simulink model "model_QK_SFSVD_ROS"  (Simulink 7.6)
settings: Solver=FixedStepDiscrete  SolverMode=SingleTasking  StartTime=0  StopTime=100  FixedStep=0.01  RelTol=1e-3
values from neighbouring files (symbols this model uses):
  parameter = block.DialogPrm(3).Data    [Kalmangain.m]    (also in init_QK_ROS.m = load('parameter'); statePrediction.m = block.DialogPrm(2).Data)
libraries: PortLib x11, simulink x2, aerolibutil x2
(part 1 of 4)
settings Model: Creator=sendobry  LastModifiedBy=sendobry
settings SolverCC: MaxConsecutiveMinStep=10
settings OptimizationCC: AccelVerboseBuild=on
settings DebuggingCC: ArrayBoundsChecking=warning  UnderspecifiedInitializationDetection=Simplified
settings RTWCC: SystemTargetFile=orocos.tlc  TemplateMakefile=orocos.tmf  Description=Linux Orocos Target  ProcessScript=orocos_make_rtw_hook
settings STFCustomTargetCC: ModelReferenceCompliant=off  GeneratePreprocessorConditionals=Disable all  MatFileLogging=on  SystemTargetFile=orocos.tlc

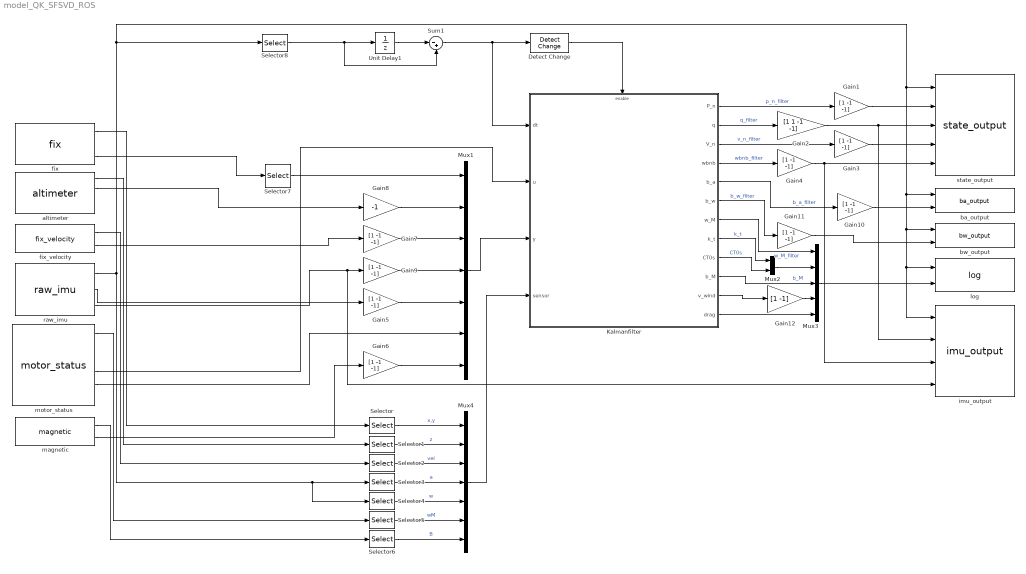
== system model_QK_SFSVD_ROS ==
  Detect Change : simulink/Logic and Bit Operations/Detect Change  SystemSampleTime=-1  vinit=0
  Gain{1,3..7,9..11} (9 alike) : Gain  Gain=[1 -1 -1]
  Gain12 : Gain  Gain=[1 -1]
  Gain2 : Gain  Gain=[1 1 -1 -1]
  Gain8 : Gain  Gain=-1
  Kalmanfilter : Subsystem
  Mux1 : Mux  Inputs=7
  Mux2 : Mux  Inputs=2
  Mux3 : Mux  Inputs=5
  Mux4 : Mux  Inputs=7
  Selector{,1..6,8} (8 alike) : Selector  InputPortWidth=2  IndexOptions=Index vector (dialog)  Indices=2  OutputSizes=1
  Selector7 : Selector  InputPortWidth=3  IndexOptions=Index vector (dialog)  Indices=[1 2]  OutputSizes=1
  Sum1 : Sum  Inputs=|-+
  Unit Delay1 : UnitDelay  SampleTime=-1
  altimeter : PortLib/altimeter  SystemSampleTime=-1
  ba_output : PortLib/ba_output  SystemSampleTime=-1
  bw_output : PortLib/bw_output  SystemSampleTime=-1
  fix : PortLib/fix  SystemSampleTime=-1
  fix_velocity : PortLib/fix_velocity  SystemSampleTime=-1
  imu_output : PortLib/imu_output  SystemSampleTime=-1
  log : PortLib/log  SystemSampleTime=-1
  magnetic : PortLib/magnetic  SystemSampleTime=-1
  motor_status : PortLib/motor_status  SystemSampleTime=-1
  raw_imu : PortLib/raw_imu  SystemSampleTime=-1
  state_output : PortLib/state_output  SystemSampleTime=-1
  wires:
  motor_status/4 -> Kalmanfilter/2(u)
  fix/3 -> Selector7/1
  altimeter/2 -> Gain8/1
  fix_velocity/2 -> Gain7/1
  raw_imu/3 -> Gain9/1, imu_output/4
  raw_imu/2 -> Gain5/1
  magnetic/2 -> Gain6/1
  Mux1/1 -> Kalmanfilter/3(y)
  Mux4/1 -> Kalmanfilter/4(sensor)
  Unit Delay1/1 -> Sum1/1
  Selector/1 -> Mux4/1  "x,y"
  Selector1/1 -> Mux4/2  "z"
  Selector2/1 -> Mux4/3  "vel"
  Selector3/1 -> Mux4/4  "a"
  Selector4/1 -> Mux4/5  "w"
  Selector5/1 -> Mux4/6  "wM"
  Selector6/1 -> Mux4/7  "B"
  fix/1 -> Selector/1
  altimeter/1 -> Selector1/1
  raw_imu/1 -> Selector3/1, Selector4/1, Selector8/1, ba_output/1, bw_output/1, log/1, imu_output/1, state_output/1
  magnetic/1 -> Selector6/1
  fix_velocity/1 -> Selector2/1
  Selector8/1 -> Sum1/2, Unit Delay1/1
  motor_status/1 -> Selector5/1
  Kalmanfilter/1(P_n) -> Gain1/1  "p_n_filter"
  Kalmanfilter/4(wbnb) -> Gain4/1  "wbnb_filter"
  Kalmanfilter/2(q) -> Gain2/1  "q_filter"
  Kalmanfilter/3(V_n) -> Gain3/1  "v_n_filter"
  Gain5/1 -> Mux1/5
  Gain6/1 -> Mux1/7
  Gain7/1 -> Mux1/3
  Gain8/1 -> Mux1/2
  Gain9/1 -> Mux1/4
  Selector7/1 -> Mux1/1
  Kalmanfilter/5(b_a) -> Gain10/1  "b_a_filter"
  Kalmanfilter/6(b_w) -> Gain11/1  "b_w_filter"
  Kalmanfilter/7(w_M) -> Mux3/1  "w_M_filter"
  Mux2/1 -> Mux3/2
  Kalmanfilter/8(k_t) -> Mux2/1  "k_t"
  Kalmanfilter/9(CT0s) -> Mux2/2  "CT0s"
  Kalmanfilter/10(b_M) -> Mux3/3  "b_M"
  Kalmanfilter/12(drag) -> Mux3/5
  Gain12/1 -> Mux3/4
  Gain1/1 -> state_output/2
  Gain2/1 -> state_output/3, imu_output/2
  Gain3/1 -> state_output/4
  Gain4/1 -> state_output/5, imu_output/3
  Gain10/1 -> ba_output/2
  Gain11/1 -> bw_output/2
  Mux3/1 -> log/2
  Kalmanfilter/11(v_wind) -> Gain12/1
  Sum1/1 -> Kalmanfilter/1(dt), Detect Change/1
  Detect Change/1 -> Kalmanfilter/Enable
  motor_status/5 -> Mux1/6

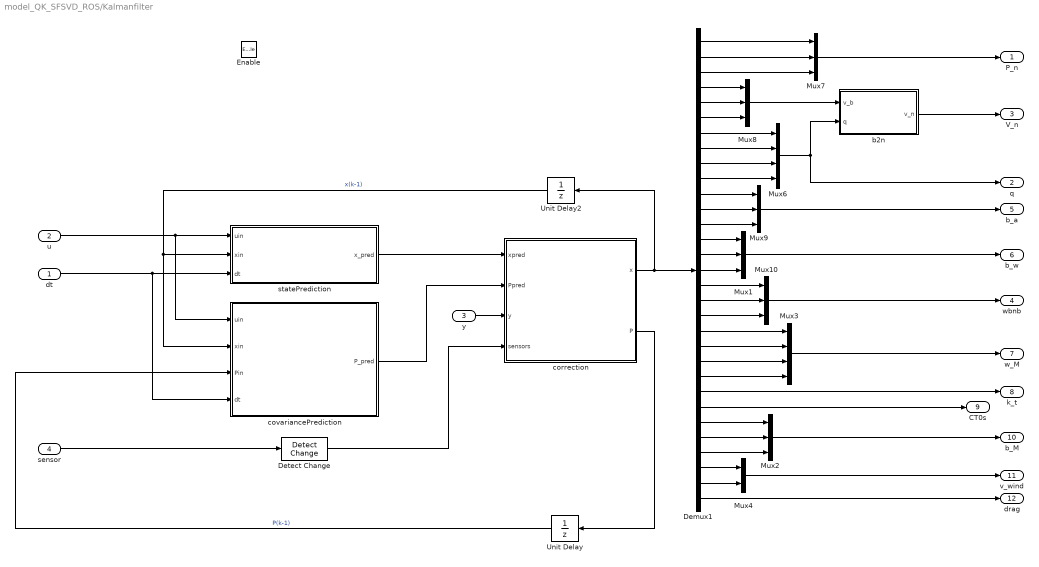
== system model_QK_SFSVD_ROS/Kalmanfilter ==
  dt : Inport
  u : Inport  Port=2
  y : Inport  Port=3
  sensor : Inport  Port=4
  Enable : EnablePort
  Demux1 : Demux  Outputs=31
  Detect Change : simulink/Logic and Bit Operations/Detect Change  SystemSampleTime=-1  vinit=0
  Mux{1..2,7..10} (6 alike) : Mux  Inputs=3
  Mux3 : Mux
  Mux4 : Mux  Inputs=2
  Mux6 : Mux
  Unit Delay : UnitDelay  X0=parameter.P0  SampleTime=-1
  Unit Delay2 : UnitDelay  X0=parameter.x0  SampleTime=-1
  b2n : Subsystem
  correction : Stateflow chart  TreatAsAtomicUnit=on
  covariancePrediction : Stateflow chart  TreatAsAtomicUnit=on
  statePrediction : Stateflow chart  TreatAsAtomicUnit=on
  P_n : Outport  InitialOutput=parameter.x0(1:3)
  q : Outport  Port=2  InitialOutput=parameter.x0(7:10)
  V_n : Outport  Port=3  InitialOutput=zeros(3,1)
  wbnb : Outport  Port=4  PortDimensions=3  InitialOutput=parameter.x0(17:19)
  b_a : Outport  Port=5  PortDimensions=3  InitialOutput=parameter.x0(11:13)
  b_w : Outport  Port=6  PortDimensions=3  InitialOutput=parameter.x0(14:16)
  w_M : Outport  Port=7  PortDimensions=4  InitialOutput=parameter.x0(20:23)
  k_t : Outport  Port=8  InitialOutput=parameter.k_t
  CT0s : Outport  Port=9  InitialOutput=parameter.CT0s
  b_M : Outport  Port=10  InitialOutput=parameter.x0(26:28)
  v_wind : Outport  Port=11  InitialOutput=parameter.x0(29:30)
  drag : Outport  Port=12  InitialOutput=parameter.x0(31)
  wires:
  Demux1/1 -> Mux7/1
  Demux1/2 -> Mux7/2
  Demux1/3 -> Mux7/3
  Demux1/20 -> Mux3/1
  Demux1/21 -> Mux3/2
  Demux1/22 -> Mux3/3
  Demux1/23 -> Mux3/4
  correction/1(x) -> Demux1/1, Unit Delay2/1
  correction/2(P) -> Unit Delay/1
  Mux6/1 -> q/1, b2n/2(q)
  Demux1/7 -> Mux6/1
  Demux1/8 -> Mux6/2
  Demux1/9 -> Mux6/3
  Demux1/10 -> Mux6/4
  u/1 -> covariancePrediction/1(uin), statePrediction/1(uin)
  Demux1/14 -> Mux1/1
  Demux1/15 -> Mux1/2
  Demux1/16 -> Mux1/3
  Demux1/4 -> Mux8/1
  Demux1/5 -> Mux8/2
  Demux1/6 -> Mux8/3
  Demux1/11 -> Mux9/1
  Demux1/12 -> Mux9/2
  Demux1/13 -> Mux9/3
  Demux1/17 -> Mux10/1
  Demux1/18 -> Mux10/2
  Demux1/19 -> Mux10/3
  Mux7/1 -> P_n/1
  Mux9/1 -> b_a/1
  Mux1/1 -> b_w/1
  Mux10/1 -> wbnb/1
  Mux3/1 -> w_M/1
  Mux2/1 -> b_M/1
  b2n/1(v_n) -> V_n/1
  Mux8/1 -> b2n/1(v_b)
  Unit Delay2/1 -> covariancePrediction/2(xin), statePrediction/2(xin)  "x(k-1)"
  Demux1/24 -> k_t/1
  Demux1/25 -> CT0s/1
  sensor/1 -> Detect Change/1
  Mux4/1 -> v_wind/1
  Demux1/31 -> drag/1
  Demux1/26 -> Mux2/1
  Demux1/27 -> Mux2/2
  Demux1/28 -> Mux2/3
  Demux1/29 -> Mux4/1
  Demux1/30 -> Mux4/2
  statePrediction/1(x_pred) -> correction/1(xpred)
  covariancePrediction/1(P_pred) -> correction/2(Ppred)
  Unit Delay/1 -> covariancePrediction/3(Pin)  "P(k-1)"
  y/1 -> correction/3(y)
  dt/1 -> covariancePrediction/4(dt), statePrediction/3(dt)
  Detect Change/1 -> correction/4(sensors)

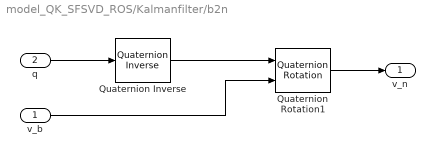
== system model_QK_SFSVD_ROS/Kalmanfilter/b2n ==
  v_b : Inport
  q : Inport  Port=2
  Quaternion Inverse : aerolibutil/Quaternion Inverse
  Quaternion Rotation1 : aerolibutil/Quaternion Rotation
  v_n : Outport
  wires:
  q/1 -> Quaternion Inverse/1
  Quaternion Rotation1/1 -> v_n/1
  Quaternion Inverse/1 -> Quaternion Rotation1/1
  v_b/1 -> Quaternion Rotation1/2
